simulink model "SIFT"  (R2015a)
settings: Solver=ode45  StartTime=0.0  StopTime=10.0  RelTol=1e-3
InitFcn:
  | %% DSPBuilder Start
  | alt_dspbuilder_update_model(bdroot)
  | %% DSPBuilder End
libraries: allblocks_alteradspbuilder2 x2272
(part 19 of 26)

== system SIFT/sift_octave1/get_descriptor/scale_space/Gaussian_scale4/Mul ==
  In00 : Inport
  In01 : Inport  Port=2
  In02 : Inport  Port=3
  In03 : Inport  Port=4
  In04 : Inport  Port=5
  In10 : Inport  Port=6
  In11 : Inport  Port=7
  In12 : Inport  Port=8
  In13 : Inport  Port=9
  In14 : Inport  Port=10
  In20 : Inport  Port=11
  In21 : Inport  Port=12
  In22 : Inport  Port=13
  In23 : Inport  Port=14
  In24 : Inport  Port=15
  In30 : Inport  Port=16
  In31 : Inport  Port=17
  In32 : Inport  Port=18
  In33 : Inport  Port=19
  In34 : Inport  Port=20
  In40 : Inport  Port=21
  In41 : Inport  Port=22
  In42 : Inport  Port=23
  In43 : Inport  Port=24
  In44 : Inport  Port=25
  clken : Inport  Port=26
  Delay : allblocks_alteradspbuilder2/Delay  pipeline=1  pipeline_display=1  ClockPhase=1  use_ena=on  use_sclr=off  allowFloatingPointOverride=on  logOutputs=off  logFile=C:\Users\ASUS\Desktop\sift_fpga\Octave_2\tb_SIFT\SIFT_sift%5Foctave1_get%5Fdescriptor_scale%5Fspace_Gaussian%5Fscale4_Mul_Delay.fixedpointlog  use_init=off  reset_value=1
  Delay1 : allblocks_alteradspbuilder2/Delay  pipeline=1  pipeline_display=1  ClockPhase=1  use_ena=on  use_sclr=off  allowFloatingPointOverride=on  logOutputs=off  logFile=C:\Users\ASUS\Desktop\sift_fpga\Octave_2\tb_SIFT\SIFT_sift%5Foctave1_get%5Fdescriptor_scale%5Fspace_Gaussian%5Fscale4_Mul_Delay1.fixedpointlog  use_init=off  reset_value=1
  Delay10 : allblocks_alteradspbuilder2/Delay  pipeline=1  pipeline_display=1  ClockPhase=1  use_ena=on  use_sclr=off  allowFloatingPointOverride=on  logOutputs=off  logFile=C:\Users\ASUS\Desktop\sift_fpga\Octave_2\tb_SIFT\SIFT_sift%5Foctave1_get%5Fdescriptor_scale%5Fspace_Gaussian%5Fscale4_Mul_Delay10.fixedpointlog  use_init=off  reset_value=1
  Delay11 : allblocks_alteradspbuilder2/Delay  pipeline=1  pipeline_display=1  ClockPhase=1  use_ena=on  use_sclr=off  allowFloatingPointOverride=on  logOutputs=off  logFile=C:\Users\ASUS\Desktop\sift_fpga\Octave_2\tb_SIFT\SIFT_sift%5Foctave1_get%5Fdescriptor_scale%5Fspace_Gaussian%5Fscale4_Mul_Delay11.fixedpointlog  use_init=off  reset_value=1
  Delay12 : allblocks_alteradspbuilder2/Delay  pipeline=1  pipeline_display=1  ClockPhase=1  use_ena=on  use_sclr=off  allowFloatingPointOverride=on  logOutputs=off  logFile=C:\Users\ASUS\Desktop\sift_fpga\Octave_2\tb_SIFT\SIFT_sift%5Foctave1_get%5Fdescriptor_scale%5Fspace_Gaussian%5Fscale4_Mul_Delay12.fixedpointlog  use_init=off  reset_value=1
  Delay13 : allblocks_alteradspbuilder2/Delay  pipeline=1  pipeline_display=1  ClockPhase=1  use_ena=on  use_sclr=off  allowFloatingPointOverride=on  logOutputs=off  logFile=C:\Users\ASUS\Desktop\sift_fpga\Octave_2\tb_SIFT\SIFT_sift%5Foctave1_get%5Fdescriptor_scale%5Fspace_Gaussian%5Fscale4_Mul_Delay13.fixedpointlog  use_init=off  reset_value=1
  Delay14 : allblocks_alteradspbuilder2/Delay  pipeline=1  pipeline_display=1  ClockPhase=1  use_ena=on  use_sclr=off  allowFloatingPointOverride=on  logOutputs=off  logFile=C:\Users\ASUS\Desktop\sift_fpga\Octave_2\tb_SIFT\SIFT_sift%5Foctave1_get%5Fdescriptor_scale%5Fspace_Gaussian%5Fscale4_Mul_Delay14.fixedpointlog  use_init=off  reset_value=1
  Delay15 : allblocks_alteradspbuilder2/Delay  pipeline=1  pipeline_display=1  ClockPhase=1  use_ena=on  use_sclr=off  allowFloatingPointOverride=on  logOutputs=off  logFile=C:\Users\ASUS\Desktop\sift_fpga\Octave_2\tb_SIFT\SIFT_sift%5Foctave1_get%5Fdescriptor_scale%5Fspace_Gaussian%5Fscale4_Mul_Delay15.fixedpointlog  use_init=off  reset_value=1
  Delay16 : allblocks_alteradspbuilder2/Delay  pipeline=1  pipeline_display=1  ClockPhase=1  use_ena=on  use_sclr=off  allowFloatingPointOverride=on  logOutputs=off  logFile=C:\Users\ASUS\Desktop\sift_fpga\Octave_2\tb_SIFT\SIFT_sift%5Foctave1_get%5Fdescriptor_scale%5Fspace_Gaussian%5Fscale4_Mul_Delay16.fixedpointlog  use_init=off  reset_value=1
  Delay17 : allblocks_alteradspbuilder2/Delay  pipeline=1  pipeline_display=1  ClockPhase=1  use_ena=on  use_sclr=off  allowFloatingPointOverride=on  logOutputs=off  logFile=C:\Users\ASUS\Desktop\sift_fpga\Octave_2\tb_SIFT\SIFT_sift%5Foctave1_get%5Fdescriptor_scale%5Fspace_Gaussian%5Fscale4_Mul_Delay17.fixedpointlog  use_init=off  reset_value=1
  Delay18 : allblocks_alteradspbuilder2/Delay  pipeline=1  pipeline_display=1  ClockPhase=1  use_ena=on  use_sclr=off  allowFloatingPointOverride=on  logOutputs=off  logFile=C:\Users\ASUS\Desktop\sift_fpga\Octave_2\tb_SIFT\SIFT_sift%5Foctave1_get%5Fdescriptor_scale%5Fspace_Gaussian%5Fscale4_Mul_Delay18.fixedpointlog  use_init=off  reset_value=1
  Delay19 : allblocks_alteradspbuilder2/Delay  pipeline=1  pipeline_display=1  ClockPhase=1  use_ena=on  use_sclr=off  allowFloatingPointOverride=on  logOutputs=off  logFile=C:\Users\ASUS\Desktop\sift_fpga\Octave_2\tb_SIFT\SIFT_sift%5Foctave1_get%5Fdescriptor_scale%5Fspace_Gaussian%5Fscale4_Mul_Delay19.fixedpointlog  use_init=off  reset_value=1
  Delay2 : allblocks_alteradspbuilder2/Delay  pipeline=1  pipeline_display=1  ClockPhase=1  use_ena=on  use_sclr=off  allowFloatingPointOverride=on  logOutputs=off  logFile=C:\Users\ASUS\Desktop\sift_fpga\Octave_2\tb_SIFT\SIFT_sift%5Foctave1_get%5Fdescriptor_scale%5Fspace_Gaussian%5Fscale4_Mul_Delay2.fixedpointlog  use_init=off  reset_value=1
  Delay20 : allblocks_alteradspbuilder2/Delay  pipeline=1  pipeline_display=1  ClockPhase=1  use_ena=on  use_sclr=off  allowFloatingPointOverride=on  logOutputs=off  logFile=C:\Users\ASUS\Desktop\sift_fpga\Octave_2\tb_SIFT\SIFT_sift%5Foctave1_get%5Fdescriptor_scale%5Fspace_Gaussian%5Fscale4_Mul_Delay20.fixedpointlog  use_init=off  reset_value=1
  Delay21 : allblocks_alteradspbuilder2/Delay  pipeline=1  pipeline_display=1  ClockPhase=1  use_ena=on  use_sclr=off  allowFloatingPointOverride=on  logOutputs=off  logFile=C:\Users\ASUS\Desktop\sift_fpga\Octave_2\tb_SIFT\SIFT_sift%5Foctave1_get%5Fdescriptor_scale%5Fspace_Gaussian%5Fscale4_Mul_Delay21.fixedpointlog  use_init=off  reset_value=1
  Delay22 : allblocks_alteradspbuilder2/Delay  pipeline=1  pipeline_display=1  ClockPhase=1  use_ena=on  use_sclr=off  allowFloatingPointOverride=on  logOutputs=off  logFile=C:\Users\ASUS\Desktop\sift_fpga\Octave_2\tb_SIFT\SIFT_sift%5Foctave1_get%5Fdescriptor_scale%5Fspace_Gaussian%5Fscale4_Mul_Delay22.fixedpointlog  use_init=off  reset_value=1
  Delay23 : allblocks_alteradspbuilder2/Delay  pipeline=1  pipeline_display=1  ClockPhase=1  use_ena=on  use_sclr=off  allowFloatingPointOverride=on  logOutputs=off  logFile=C:\Users\ASUS\Desktop\sift_fpga\Octave_2\tb_SIFT\SIFT_sift%5Foctave1_get%5Fdescriptor_scale%5Fspace_Gaussian%5Fscale4_Mul_Delay23.fixedpointlog  use_init=off  reset_value=1
  Delay24 : allblocks_alteradspbuilder2/Delay  pipeline=1  pipeline_display=1  ClockPhase=1  use_ena=on  use_sclr=off  allowFloatingPointOverride=on  logOutputs=off  logFile=C:\Users\ASUS\Desktop\sift_fpga\Octave_2\tb_SIFT\SIFT_sift%5Foctave1_get%5Fdescriptor_scale%5Fspace_Gaussian%5Fscale4_Mul_Delay24.fixedpointlog  use_init=off  reset_value=1
  Delay3 : allblocks_alteradspbuilder2/Delay  pipeline=1  pipeline_display=1  ClockPhase=1  use_ena=on  use_sclr=off  allowFloatingPointOverride=on  logOutputs=off  logFile=C:\Users\ASUS\Desktop\sift_fpga\Octave_2\tb_SIFT\SIFT_sift%5Foctave1_get%5Fdescriptor_scale%5Fspace_Gaussian%5Fscale4_Mul_Delay3.fixedpointlog  use_init=off  reset_value=1
  Delay4 : allblocks_alteradspbuilder2/Delay  pipeline=1  pipeline_display=1  ClockPhase=1  use_ena=on  use_sclr=off  allowFloatingPointOverride=on  logOutputs=off  logFile=C:\Users\ASUS\Desktop\sift_fpga\Octave_2\tb_SIFT\SIFT_sift%5Foctave1_get%5Fdescriptor_scale%5Fspace_Gaussian%5Fscale4_Mul_Delay4.fixedpointlog  use_init=off  reset_value=1
  Delay5 : allblocks_alteradspbuilder2/Delay  pipeline=1  pipeline_display=1  ClockPhase=1  use_ena=on  use_sclr=off  allowFloatingPointOverride=on  logOutputs=off  logFile=C:\Users\ASUS\Desktop\sift_fpga\Octave_2\tb_SIFT\SIFT_sift%5Foctave1_get%5Fdescriptor_scale%5Fspace_Gaussian%5Fscale4_Mul_Delay5.fixedpointlog  use_init=off  reset_value=1
  Delay6 : allblocks_alteradspbuilder2/Delay  pipeline=1  pipeline_display=1  ClockPhase=1  use_ena=on  use_sclr=off  allowFloatingPointOverride=on  logOutputs=off  logFile=C:\Users\ASUS\Desktop\sift_fpga\Octave_2\tb_SIFT\SIFT_sift%5Foctave1_get%5Fdescriptor_scale%5Fspace_Gaussian%5Fscale4_Mul_Delay6.fixedpointlog  use_init=off  reset_value=1
  Delay7 : allblocks_alteradspbuilder2/Delay  pipeline=1  pipeline_display=1  ClockPhase=1  use_ena=on  use_sclr=off  allowFloatingPointOverride=on  logOutputs=off  logFile=C:\Users\ASUS\Desktop\sift_fpga\Octave_2\tb_SIFT\SIFT_sift%5Foctave1_get%5Fdescriptor_scale%5Fspace_Gaussian%5Fscale4_Mul_Delay7.fixedpointlog  use_init=off  reset_value=1
  Delay8 : allblocks_alteradspbuilder2/Delay  pipeline=1  pipeline_display=1  ClockPhase=1  use_ena=on  use_sclr=off  allowFloatingPointOverride=on  logOutputs=off  logFile=C:\Users\ASUS\Desktop\sift_fpga\Octave_2\tb_SIFT\SIFT_sift%5Foctave1_get%5Fdescriptor_scale%5Fspace_Gaussian%5Fscale4_Mul_Delay8.fixedpointlog  use_init=off  reset_value=1
  Delay9 : allblocks_alteradspbuilder2/Delay  pipeline=1  pipeline_display=1  ClockPhase=1  use_ena=on  use_sclr=off  allowFloatingPointOverride=on  logOutputs=off  logFile=C:\Users\ASUS\Desktop\sift_fpga\Octave_2\tb_SIFT\SIFT_sift%5Foctave1_get%5Fdescriptor_scale%5Fspace_Gaussian%5Fscale4_Mul_Delay9.fixedpointlog  use_init=off  reset_value=1
  Gain : allblocks_alteradspbuilder2/Gain  vgain=0.0232  BusType=Unsigned Fractional  bwl=8  bwr=16  pipeline=16  pipeline_display=16  allowFloatingPointOverride=on  logOutputs=off  logFile=C:\Users\ASUS\Desktop\sift_fpga\Octave_2\tb_SIFT\SIFT_sift%5Foctave1_get%5Fdescriptor_scale%5Fspace_Gaussian%5Fscale4_Mul_Gain.fixedpointlog  use_ena=on  use_aclr=off  lpm=off  MaskValue=1
  Gain1 : allblocks_alteradspbuilder2/Gain  vgain=0.0338  BusType=Unsigned Fractional  bwl=8  bwr=16  pipeline=16  pipeline_display=16  allowFloatingPointOverride=on  logOutputs=off  logFile=C:\Users\ASUS\Desktop\sift_fpga\Octave_2\tb_SIFT\SIFT_sift%5Foctave1_get%5Fdescriptor_scale%5Fspace_Gaussian%5Fscale4_Mul_Gain1.fixedpointlog  use_ena=on  use_aclr=off  lpm=off  MaskValue=1
  Gain10 : allblocks_alteradspbuilder2/Gain  vgain=0.0383  BusType=Unsigned Fractional  bwl=8  bwr=16  pipeline=16  pipeline_display=16  allowFloatingPointOverride=on  logOutputs=off  logFile=C:\Users\ASUS\Desktop\sift_fpga\Octave_2\tb_SIFT\SIFT_sift%5Foctave1_get%5Fdescriptor_scale%5Fspace_Gaussian%5Fscale4_Mul_Gain10.fixedpointlog  use_ena=on  use_aclr=off  lpm=off  MaskValue=1
  Gain11 : allblocks_alteradspbuilder2/Gain  vgain=0.0558  BusType=Unsigned Fractional  bwl=8  bwr=16  pipeline=16  pipeline_display=16  allowFloatingPointOverride=on  logOutputs=off  logFile=C:\Users\ASUS\Desktop\sift_fpga\Octave_2\tb_SIFT\SIFT_sift%5Foctave1_get%5Fdescriptor_scale%5Fspace_Gaussian%5Fscale4_Mul_Gain11.fixedpointlog  use_ena=on  use_aclr=off  lpm=off  MaskValue=1
  Gain12 : allblocks_alteradspbuilder2/Gain  vgain=0.0632  BusType=Unsigned Fractional  bwl=8  bwr=16  pipeline=16  pipeline_display=16  allowFloatingPointOverride=on  logOutputs=off  logFile=C:\Users\ASUS\Desktop\sift_fpga\Octave_2\tb_SIFT\SIFT_sift%5Foctave1_get%5Fdescriptor_scale%5Fspace_Gaussian%5Fscale4_Mul_Gain12.fixedpointlog  use_ena=on  use_aclr=off  lpm=off  MaskValue=1
  Gain13 : allblocks_alteradspbuilder2/Gain  vgain=0.0558  BusType=Unsigned Fractional  bwl=8  bwr=16  pipeline=16  pipeline_display=16  allowFloatingPointOverride=on  logOutputs=off  logFile=C:\Users\ASUS\Desktop\sift_fpga\Octave_2\tb_SIFT\SIFT_sift%5Foctave1_get%5Fdescriptor_scale%5Fspace_Gaussian%5Fscale4_Mul_Gain13.fixedpointlog  use_ena=on  use_aclr=off  lpm=off  MaskValue=1
  Gain14 : allblocks_alteradspbuilder2/Gain  vgain=0.0383  BusType=Unsigned Fractional  bwl=8  bwr=16  pipeline=16  pipeline_display=16  allowFloatingPointOverride=on  logOutputs=off  logFile=C:\Users\ASUS\Desktop\sift_fpga\Octave_2\tb_SIFT\SIFT_sift%5Foctave1_get%5Fdescriptor_scale%5Fspace_Gaussian%5Fscale4_Mul_Gain14.fixedpointlog  use_ena=on  use_aclr=off  lpm=off  MaskValue=1
  Gain15 : allblocks_alteradspbuilder2/Gain  vgain=0.0338  BusType=Unsigned Fractional  bwl=8  bwr=16  pipeline=16  pipeline_display=16  allowFloatingPointOverride=on  logOutputs=off  logFile=C:\Users\ASUS\Desktop\sift_fpga\Octave_2\tb_SIFT\SIFT_sift%5Foctave1_get%5Fdescriptor_scale%5Fspace_Gaussian%5Fscale4_Mul_Gain15.fixedpointlog  use_ena=on  use_aclr=off  lpm=off  MaskValue=1
  Gain16 : allblocks_alteradspbuilder2/Gain  vgain=0.0492  BusType=Unsigned Fractional  bwl=8  bwr=16  pipeline=16  pipeline_display=16  allowFloatingPointOverride=on  logOutputs=off  logFile=C:\Users\ASUS\Desktop\sift_fpga\Octave_2\tb_SIFT\SIFT_sift%5Foctave1_get%5Fdescriptor_scale%5Fspace_Gaussian%5Fscale4_Mul_Gain16.fixedpointlog  use_ena=on  use_aclr=off  lpm=off  MaskValue=1
  Gain17 : allblocks_alteradspbuilder2/Gain  vgain=0.0558  BusType=Unsigned Fractional  bwl=8  bwr=16  pipeline=16  pipeline_display=16  allowFloatingPointOverride=on  logOutputs=off  logFile=C:\Users\ASUS\Desktop\sift_fpga\Octave_2\tb_SIFT\SIFT_sift%5Foctave1_get%5Fdescriptor_scale%5Fspace_Gaussian%5Fscale4_Mul_Gain17.fixedpointlog  use_ena=on  use_aclr=off  lpm=off  MaskValue=1
  Gain18 : allblocks_alteradspbuilder2/Gain  vgain=0.0492  BusType=Unsigned Fractional  bwl=8  bwr=16  pipeline=16  pipeline_display=16  allowFloatingPointOverride=on  logOutputs=off  logFile=C:\Users\ASUS\Desktop\sift_fpga\Octave_2\tb_SIFT\SIFT_sift%5Foctave1_get%5Fdescriptor_scale%5Fspace_Gaussian%5Fscale4_Mul_Gain18.fixedpointlog  use_ena=on  use_aclr=off  lpm=off  MaskValue=1
  Gain19 : allblocks_alteradspbuilder2/Gain  vgain=0.0338  BusType=Unsigned Fractional  bwl=8  bwr=16  pipeline=16  pipeline_display=16  allowFloatingPointOverride=on  logOutputs=off  logFile=C:\Users\ASUS\Desktop\sift_fpga\Octave_2\tb_SIFT\SIFT_sift%5Foctave1_get%5Fdescriptor_scale%5Fspace_Gaussian%5Fscale4_Mul_Gain19.fixedpointlog  use_ena=on  use_aclr=off  lpm=off  MaskValue=1
  Gain2 : allblocks_alteradspbuilder2/Gain  vgain=0.0383  BusType=Unsigned Fractional  bwl=8  bwr=16  pipeline=16  pipeline_display=16  allowFloatingPointOverride=on  logOutputs=off  logFile=C:\Users\ASUS\Desktop\sift_fpga\Octave_2\tb_SIFT\SIFT_sift%5Foctave1_get%5Fdescriptor_scale%5Fspace_Gaussian%5Fscale4_Mul_Gain2.fixedpointlog  use_ena=on  use_aclr=off  lpm=off  MaskValue=1
  Gain20 : allblocks_alteradspbuilder2/Gain  vgain=0.0232  BusType=Unsigned Fractional  bwl=8  bwr=16  pipeline=16  pipeline_display=16  allowFloatingPointOverride=on  logOutputs=off  logFile=C:\Users\ASUS\Desktop\sift_fpga\Octave_2\tb_SIFT\SIFT_sift%5Foctave1_get%5Fdescriptor_scale%5Fspace_Gaussian%5Fscale4_Mul_Gain20.fixedpointlog  use_ena=on  use_aclr=off  lpm=off  MaskValue=1
  Gain21 : allblocks_alteradspbuilder2/Gain  vgain=0.0338  BusType=Unsigned Fractional  bwl=8  bwr=16  pipeline=16  pipeline_display=16  allowFloatingPointOverride=on  logOutputs=off  logFile=C:\Users\ASUS\Desktop\sift_fpga\Octave_2\tb_SIFT\SIFT_sift%5Foctave1_get%5Fdescriptor_scale%5Fspace_Gaussian%5Fscale4_Mul_Gain21.fixedpointlog  use_ena=on  use_aclr=off  lpm=off  MaskValue=1
  Gain22 : allblocks_alteradspbuilder2/Gain  vgain=0.0383  BusType=Unsigned Fractional  bwl=8  bwr=16  pipeline=16  pipeline_display=16  allowFloatingPointOverride=on  logOutputs=off  logFile=C:\Users\ASUS\Desktop\sift_fpga\Octave_2\tb_SIFT\SIFT_sift%5Foctave1_get%5Fdescriptor_scale%5Fspace_Gaussian%5Fscale4_Mul_Gain22.fixedpointlog  use_ena=on  use_aclr=off  lpm=off  MaskValue=1
  Gain23 : allblocks_alteradspbuilder2/Gain  vgain=0.0338  BusType=Unsigned Fractional  bwl=8  bwr=16  pipeline=16  pipeline_display=16  allowFloatingPointOverride=on  logOutputs=off  logFile=C:\Users\ASUS\Desktop\sift_fpga\Octave_2\tb_SIFT\SIFT_sift%5Foctave1_get%5Fdescriptor_scale%5Fspace_Gaussian%5Fscale4_Mul_Gain23.fixedpointlog  use_ena=on  use_aclr=off  lpm=off  MaskValue=1
  Gain24 : allblocks_alteradspbuilder2/Gain  vgain=0.0232  BusType=Unsigned Fractional  bwl=8  bwr=16  pipeline=16  pipeline_display=16  allowFloatingPointOverride=on  logOutputs=off  logFile=C:\Users\ASUS\Desktop\sift_fpga\Octave_2\tb_SIFT\SIFT_sift%5Foctave1_get%5Fdescriptor_scale%5Fspace_Gaussian%5Fscale4_Mul_Gain24.fixedpointlog  use_ena=on  use_aclr=off  lpm=off  MaskValue=1
  Gain3 : allblocks_alteradspbuilder2/Gain  vgain=0.0338  BusType=Unsigned Fractional  bwl=8  bwr=16  pipeline=16  pipeline_display=16  allowFloatingPointOverride=on  logOutputs=off  logFile=C:\Users\ASUS\Desktop\sift_fpga\Octave_2\tb_SIFT\SIFT_sift%5Foctave1_get%5Fdescriptor_scale%5Fspace_Gaussian%5Fscale4_Mul_Gain3.fixedpointlog  use_ena=on  use_aclr=off  lpm=off  MaskValue=1
  Gain4 : allblocks_alteradspbuilder2/Gain  vgain=0.0232  BusType=Unsigned Fractional  bwl=8  bwr=16  pipeline=16  pipeline_display=16  allowFloatingPointOverride=on  logOutputs=off  logFile=C:\Users\ASUS\Desktop\sift_fpga\Octave_2\tb_SIFT\SIFT_sift%5Foctave1_get%5Fdescriptor_scale%5Fspace_Gaussian%5Fscale4_Mul_Gain4.fixedpointlog  use_ena=on  use_aclr=off  lpm=off  MaskValue=1
  Gain5 : allblocks_alteradspbuilder2/Gain  vgain=0.0338  BusType=Unsigned Fractional  bwl=8  bwr=16  pipeline=16  pipeline_display=16  allowFloatingPointOverride=on  logOutputs=off  logFile=C:\Users\ASUS\Desktop\sift_fpga\Octave_2\tb_SIFT\SIFT_sift%5Foctave1_get%5Fdescriptor_scale%5Fspace_Gaussian%5Fscale4_Mul_Gain5.fixedpointlog  use_ena=on  use_aclr=off  lpm=off  MaskValue=1
  Gain6 : allblocks_alteradspbuilder2/Gain  vgain=0.0492  BusType=Unsigned Fractional  bwl=8  bwr=16  pipeline=16  pipeline_display=16  allowFloatingPointOverride=on  logOutputs=off  logFile=C:\Users\ASUS\Desktop\sift_fpga\Octave_2\tb_SIFT\SIFT_sift%5Foctave1_get%5Fdescriptor_scale%5Fspace_Gaussian%5Fscale4_Mul_Gain6.fixedpointlog  use_ena=on  use_aclr=off  lpm=off  MaskValue=1
  Gain7 : allblocks_alteradspbuilder2/Gain  vgain=0.0558  BusType=Unsigned Fractional  bwl=8  bwr=16  pipeline=16  pipeline_display=16  allowFloatingPointOverride=on  logOutputs=off  logFile=C:\Users\ASUS\Desktop\sift_fpga\Octave_2\tb_SIFT\SIFT_sift%5Foctave1_get%5Fdescriptor_scale%5Fspace_Gaussian%5Fscale4_Mul_Gain7.fixedpointlog  use_ena=on  use_aclr=off  lpm=off  MaskValue=1
  Gain8 : allblocks_alteradspbuilder2/Gain  vgain=0.0492  BusType=Unsigned Fractional  bwl=8  bwr=16  pipeline=16  pipeline_display=16  allowFloatingPointOverride=on  logOutputs=off  logFile=C:\Users\ASUS\Desktop\sift_fpga\Octave_2\tb_SIFT\SIFT_sift%5Foctave1_get%5Fdescriptor_scale%5Fspace_Gaussian%5Fscale4_Mul_Gain8.fixedpointlog  use_ena=on  use_aclr=off  lpm=off  MaskValue=1
  Gain9 : allblocks_alteradspbuilder2/Gain  vgain=0.0338  BusType=Unsigned Fractional  bwl=8  bwr=16  pipeline=16  pipeline_display=16  allowFloatingPointOverride=on  logOutputs=off  logFile=C:\Users\ASUS\Desktop\sift_fpga\Octave_2\tb_SIFT\SIFT_sift%5Foctave1_get%5Fdescriptor_scale%5Fspace_Gaussian%5Fscale4_Mul_Gain9.fixedpointlog  use_ena=on  use_aclr=off  lpm=off  MaskValue=1
  Parallel Adder Subtractor : allblocks_alteradspbuilder2/Parallel Adder Subtractor  number_of_inputs=25  direction=+  use_pipeline=on  pipeline_display=5  phase_selection=1  use_ena=on  use_aclr=off  allowFloatingPointOverride=on  logOutputs=off  logFile=C:\Users\ASUS\Desktop\sift_fpga\Octave_2\tb_SIFT\SIFT_sift%5Foctave1_get%5Fdescriptor_scale%5Fspace_Gaussian%5Fscale4_Mul_Parallel+Adder+Subtractor.fixedpointlog
  pixel : Outport
  wires:
  In00/1 -> [data_00]
  In21/1 -> [data_21]
  In30/1 -> [data_30]
  In04/1 -> [data_04]
  In03/1 -> [data_03]
  In14/1 -> [data_14]
  In02/1 -> [data_02]
  In13/1 -> [data_13]
  In31/1 -> [data_31]
  In20/1 -> [data_20]
  In22/1 -> [data_22]
  In24/1 -> [data_24]
  In23/1 -> [data_23]
  In01/1 -> [data_01]
  In32/1 -> [data_32]
  In34/1 -> [data_34]
  In33/1 -> [data_33]
  In40/1 -> [data_40]
  In41/1 -> [data_41]
  In42/1 -> [data_42]
  In44/1 -> [data_44]
  In12/1 -> [data_12]
  In11/1 -> [data_11]
  In10/1 -> [data_10]
  Delay1/1 -> [mul_01]
  Delay4/1 -> [mul_04]
  [clken] -> Delay1/2, Gain1/2
  [data_11] -> Gain6/1
  Delay6/1 -> [mul_11]
  [data_12] -> Gain7/1
  [clken] -> Delay4/2, Gain4/2
  Delay2/1 -> [mul_02]
  [data_01] -> Gain1/1
  [data_04] -> Gain4/1
  Gain2/1 -> Delay2/1
  [clken] -> Delay6/2, Gain6/2
  Delay3/1 -> [mul_03]
  clken/1 -> [clken]
  [clken] -> Delay7/2, Gain7/2
  [data_02] -> Gain2/1
  Gain7/1 -> Delay7/1
  Gain1/1 -> Delay1/1
  [data_03] -> Gain3/1
  [data_00] -> Gain/1
  Gain5/1 -> Delay5/1
  Gain6/1 -> Delay6/1
  Delay5/1 -> [mul_10]
  Gain4/1 -> Delay4/1
  Gain/1 -> Delay/1
  Delay/1 -> [mul_00]
  [clken] -> Delay3/2, Gain3/2
  Gain3/1 -> Delay3/1
  [data_10] -> Gain5/1
  In43/1 -> [data_43]
  [clken] -> Delay2/2, Gain2/2
  [clken] -> Delay5/2, Gain5/2
  [clken] -> Delay13/2, Gain13/2
  [clken] -> Delay15/2, Gain15/2
  [data_22] -> Gain12/1
  [clken] -> Delay8/2, Gain8/2
  [data_20] -> Gain10/1
  [clken] -> Delay9/2, Gain9/2
  Delay9/1 -> [mul_14]
  Gain9/1 -> Delay9/1
  Delay10/1 -> [mul_20]
  [clken] -> Delay11/2, Gain11/2
  Delay11/1 -> [mul_21]
  [clken] -> Delay10/2, Gain10/2
  Gain10/1 -> Delay10/1
  Gain12/1 -> Delay12/1
  [data_14] -> Gain9/1
  Delay13/1 -> [mul_23]
  [clken] -> Delay14/2, Gain14/2
  Gain14/1 -> Delay14/1
  Delay7/1 -> [mul_12]
  [data_13] -> Gain8/1
  Gain15/1 -> Delay15/1
  [clken] -> Delay12/2, Gain12/2
  Gain13/1 -> Delay13/1
  Delay8/1 -> [mul_13]
  Delay12/1 -> [mul_22]
  [data_24] -> Gain14/1
  Gain11/1 -> Delay11/1
  [data_23] -> Gain13/1
  Delay14/1 -> [mul_24]
  Gain8/1 -> Delay8/1
  [data_30] -> Gain15/1
  [data_21] -> Gain11/1
  Gain18/1 -> Delay18/1
  Gain23/1 -> Delay23/1
  Gain16/1 -> Delay16/1
  Delay16/1 -> [mul_31]
  [data_34] -> Gain19/1
  [clken] -> Delay20/2, Gain20/2
  [clken] -> Delay19/2, Gain19/2
  Gain17/1 -> Delay17/1
  Delay17/1 -> [mul_32]
  Delay18/1 -> [mul_33]
  Gain20/1 -> Delay20/1
  Delay20/1 -> [mul_40]
  [clken] -> Delay17/2, Gain17/2
  [clken] -> Delay21/2, Gain21/2
  [data_31] -> Gain16/1
  [data_33] -> Gain18/1
  [clken] -> Delay16/2, Gain16/2
  Delay19/1 -> [mul_34]
  Gain21/1 -> Delay21/1
  [data_42] -> Gain22/1
  Delay21/1 -> [mul_41]
  Delay22/1 -> [mul_42]
  [data_43] -> Gain23/1
  [clken] -> Delay23/2, Gain23/2
  Delay15/1 -> [mul_30]
  [clken] -> Delay18/2, Gain18/2
  Gain19/1 -> Delay19/1
  Gain22/1 -> Delay22/1
  [data_40] -> Gain20/1
  [data_32] -> Gain17/1
  [data_41] -> Gain21/1
  [clken] -> Delay22/2, Gain22/2
  Delay24/1 -> [mul_44]
  Gain24/1 -> Delay24/1
  [clken] -> Delay24/2, Gain24/2
  [data_44] -> Gain24/1
  Delay23/1 -> [mul_43]
  [clken] -> Delay/2, Gain/2
  [pixel] -> pixel/1
  [mul_00] -> Parallel Adder Subtractor/1
  [mul_01] -> Parallel Adder Subtractor/2
  [mul_02] -> Parallel Adder Subtractor/3
  [mul_03] -> Parallel Adder Subtractor/4
  [mul_04] -> Parallel Adder Subtractor/5
  [mul_10] -> Parallel Adder Subtractor/6
  [mul_11] -> Parallel Adder Subtractor/7
  [mul_12] -> Parallel Adder Subtractor/8
  [mul_13] -> Parallel Adder Subtractor/9
  [mul_14] -> Parallel Adder Subtractor/10
  [mul_20] -> Parallel Adder Subtractor/11
  [mul_21] -> Parallel Adder Subtractor/12
  [mul_22] -> Parallel Adder Subtractor/13
  [mul_23] -> Parallel Adder Subtractor/14
  [mul_24] -> Parallel Adder Subtractor/15
  [mul_31] -> Parallel Adder Subtractor/17
  [mul_32] -> Parallel Adder Subtractor/18
  [mul_33] -> Parallel Adder Subtractor/19
  [mul_34] -> Parallel Adder Subtractor/20
  [mul_40] -> Parallel Adder Subtractor/21
  [mul_41] -> Parallel Adder Subtractor/22
  [mul_42] -> Parallel Adder Subtractor/23
  [mul_43] -> Parallel Adder Subtractor/24
  [mul_44] -> Parallel Adder Subtractor/25
  [mul_30] -> Parallel Adder Subtractor/16
  [clken] -> Parallel Adder Subtractor/26
  Parallel Adder Subtractor/1 -> [pixel]

== system SIFT/sift_octave1/get_descriptor/scale_space/Gaussian_scale4/line_buff ==
  dataIn : Inport
  clken : Inport  Port=2
  Delay : allblocks_alteradspbuilder2/Delay  pipeline=1  pipeline_display=1  ClockPhase=1  use_ena=on  use_sclr=off  allowFloatingPointOverride=on  logOutputs=off  logFile=C:\Users\ASUS\Desktop\sift_fpga\Octave_2\tb_SIFT\SIFT_sift%5Foctave1_get%5Fdescriptor_scale%5Fspace_Gaussian%5Fscale4_line%5Fbuff_Delay.fixedpointlog  use_init=off  reset_value=1
  Delay1 : allblocks_alteradspbuilder2/Delay  pipeline=1  pipeline_display=1  ClockPhase=1  use_ena=on  use_sclr=off  allowFloatingPointOverride=on  logOutputs=off  logFile=C:\Users\ASUS\Desktop\sift_fpga\Octave_2\tb_SIFT\SIFT_sift%5Foctave1_get%5Fdescriptor_scale%5Fspace_Gaussian%5Fscale4_line%5Fbuff_Delay1.fixedpointlog  use_init=off  reset_value=1
  Delay10 : allblocks_alteradspbuilder2/Delay  pipeline=1  pipeline_display=1  ClockPhase=1  use_ena=on  use_sclr=off  allowFloatingPointOverride=on  logOutputs=off  logFile=C:\Users\ASUS\Desktop\sift_fpga\Octave_2\tb_SIFT\SIFT_sift%5Foctave1_get%5Fdescriptor_scale%5Fspace_Gaussian%5Fscale4_line%5Fbuff_Delay10.fixedpointlog  use_init=off  reset_value=1
  Delay11 : allblocks_alteradspbuilder2/Delay  pipeline=1  pipeline_display=1  ClockPhase=1  use_ena=on  use_sclr=off  allowFloatingPointOverride=on  logOutputs=off  logFile=C:\Users\ASUS\Desktop\sift_fpga\Octave_2\tb_SIFT\SIFT_sift%5Foctave1_get%5Fdescriptor_scale%5Fspace_Gaussian%5Fscale4_line%5Fbuff_Delay11.fixedpointlog  use_init=off  reset_value=1
  Delay12 : allblocks_alteradspbuilder2/Delay  pipeline=1  pipeline_display=1  ClockPhase=1  use_ena=on  use_sclr=off  allowFloatingPointOverride=on  logOutputs=off  logFile=C:\Users\ASUS\Desktop\sift_fpga\Octave_2\tb_SIFT\SIFT_sift%5Foctave1_get%5Fdescriptor_scale%5Fspace_Gaussian%5Fscale4_line%5Fbuff_Delay12.fixedpointlog  use_init=off  reset_value=1
  Delay13 : allblocks_alteradspbuilder2/Delay  pipeline=1  pipeline_display=1  ClockPhase=1  use_ena=on  use_sclr=off  allowFloatingPointOverride=on  logOutputs=off  logFile=C:\Users\ASUS\Desktop\sift_fpga\Octave_2\tb_SIFT\SIFT_sift%5Foctave1_get%5Fdescriptor_scale%5Fspace_Gaussian%5Fscale4_line%5Fbuff_Delay13.fixedpointlog  use_init=off  reset_value=1
  Delay14 : allblocks_alteradspbuilder2/Delay  pipeline=1  pipeline_display=1  ClockPhase=1  use_ena=on  use_sclr=off  allowFloatingPointOverride=on  logOutputs=off  logFile=C:\Users\ASUS\Desktop\sift_fpga\Octave_2\tb_SIFT\SIFT_sift%5Foctave1_get%5Fdescriptor_scale%5Fspace_Gaussian%5Fscale4_line%5Fbuff_Delay14.fixedpointlog  use_init=off  reset_value=1
  Delay15 : allblocks_alteradspbuilder2/Delay  pipeline=1  pipeline_display=1  ClockPhase=1  use_ena=on  use_sclr=off  allowFloatingPointOverride=on  logOutputs=off  logFile=C:\Users\ASUS\Desktop\sift_fpga\Octave_2\tb_SIFT\SIFT_sift%5Foctave1_get%5Fdescriptor_scale%5Fspace_Gaussian%5Fscale4_line%5Fbuff_Delay15.fixedpointlog  use_init=off  reset_value=1
  Delay16 : allblocks_alteradspbuilder2/Delay  pipeline=1  pipeline_display=1  ClockPhase=1  use_ena=on  use_sclr=off  allowFloatingPointOverride=on  logOutputs=off  logFile=C:\Users\ASUS\Desktop\sift_fpga\Octave_2\tb_SIFT\SIFT_sift%5Foctave1_get%5Fdescriptor_scale%5Fspace_Gaussian%5Fscale4_line%5Fbuff_Delay16.fixedpointlog  use_init=off  reset_value=1
  Delay17 : allblocks_alteradspbuilder2/Delay  pipeline=1  pipeline_display=1  ClockPhase=1  use_ena=on  use_sclr=off  allowFloatingPointOverride=on  logOutputs=off  logFile=C:\Users\ASUS\Desktop\sift_fpga\Octave_2\tb_SIFT\SIFT_sift%5Foctave1_get%5Fdescriptor_scale%5Fspace_Gaussian%5Fscale4_line%5Fbuff_Delay17.fixedpointlog  use_init=off  reset_value=1
  Delay18 : allblocks_alteradspbuilder2/Delay  pipeline=1  pipeline_display=1  ClockPhase=1  use_ena=on  use_sclr=off  allowFloatingPointOverride=on  logOutputs=off  logFile=C:\Users\ASUS\Desktop\sift_fpga\Octave_2\tb_SIFT\SIFT_sift%5Foctave1_get%5Fdescriptor_scale%5Fspace_Gaussian%5Fscale4_line%5Fbuff_Delay18.fixedpointlog  use_init=off  reset_value=1
  Delay19 : allblocks_alteradspbuilder2/Delay  pipeline=1  pipeline_display=1  ClockPhase=1  use_ena=on  use_sclr=off  allowFloatingPointOverride=on  logOutputs=off  logFile=C:\Users\ASUS\Desktop\sift_fpga\Octave_2\tb_SIFT\SIFT_sift%5Foctave1_get%5Fdescriptor_scale%5Fspace_Gaussian%5Fscale4_line%5Fbuff_Delay19.fixedpointlog  use_init=off  reset_value=1
  Delay2 : allblocks_alteradspbuilder2/Delay  pipeline=1  pipeline_display=1  ClockPhase=1  use_ena=on  use_sclr=off  allowFloatingPointOverride=on  logOutputs=off  logFile=C:\Users\ASUS\Desktop\sift_fpga\Octave_2\tb_SIFT\SIFT_sift%5Foctave1_get%5Fdescriptor_scale%5Fspace_Gaussian%5Fscale4_line%5Fbuff_Delay2.fixedpointlog  use_init=off  reset_value=1
  Delay20 : allblocks_alteradspbuilder2/Delay  pipeline=1  pipeline_display=1  ClockPhase=1  use_ena=on  use_sclr=off  allowFloatingPointOverride=on  logOutputs=off  logFile=C:\Users\ASUS\Desktop\sift_fpga\Octave_2\tb_SIFT\SIFT_sift%5Foctave1_get%5Fdescriptor_scale%5Fspace_Gaussian%5Fscale4_line%5Fbuff_Delay20.fixedpointlog  use_init=off  reset_value=1
  Delay3 : allblocks_alteradspbuilder2/Delay  pipeline=1  pipeline_display=1  ClockPhase=1  use_ena=on  use_sclr=off  allowFloatingPointOverride=on  logOutputs=off  logFile=C:\Users\ASUS\Desktop\sift_fpga\Octave_2\tb_SIFT\SIFT_sift%5Foctave1_get%5Fdescriptor_scale%5Fspace_Gaussian%5Fscale4_line%5Fbuff_Delay3.fixedpointlog  use_init=off  reset_value=1
  Delay4 : allblocks_alteradspbuilder2/Delay  pipeline=1  pipeline_display=1  ClockPhase=1  use_ena=on  use_sclr=off  allowFloatingPointOverride=on  logOutputs=off  logFile=C:\Users\ASUS\Desktop\sift_fpga\Octave_2\tb_SIFT\SIFT_sift%5Foctave1_get%5Fdescriptor_scale%5Fspace_Gaussian%5Fscale4_line%5Fbuff_Delay4.fixedpointlog  use_init=off  reset_value=1
  Delay5 : allblocks_alteradspbuilder2/Delay  pipeline=1  pipeline_display=1  ClockPhase=1  use_ena=on  use_sclr=off  allowFloatingPointOverride=on  logOutputs=off  logFile=C:\Users\ASUS\Desktop\sift_fpga\Octave_2\tb_SIFT\SIFT_sift%5Foctave1_get%5Fdescriptor_scale%5Fspace_Gaussian%5Fscale4_line%5Fbuff_Delay5.fixedpointlog  use_init=off  reset_value=1
  Delay6 : allblocks_alteradspbuilder2/Delay  pipeline=1  pipeline_display=1  ClockPhase=1  use_ena=on  use_sclr=off  allowFloatingPointOverride=on  logOutputs=off  logFile=C:\Users\ASUS\Desktop\sift_fpga\Octave_2\tb_SIFT\SIFT_sift%5Foctave1_get%5Fdescriptor_scale%5Fspace_Gaussian%5Fscale4_line%5Fbuff_Delay6.fixedpointlog  use_init=off  reset_value=1
  Delay7 : allblocks_alteradspbuilder2/Delay  pipeline=1  pipeline_display=1  ClockPhase=1  use_ena=on  use_sclr=off  allowFloatingPointOverride=on  logOutputs=off  logFile=C:\Users\ASUS\Desktop\sift_fpga\Octave_2\tb_SIFT\SIFT_sift%5Foctave1_get%5Fdescriptor_scale%5Fspace_Gaussian%5Fscale4_line%5Fbuff_Delay7.fixedpointlog  use_init=off  reset_value=1
  Delay8 : allblocks_alteradspbuilder2/Delay  pipeline=1  pipeline_display=1  ClockPhase=1  use_ena=on  use_sclr=off  allowFloatingPointOverride=on  logOutputs=off  logFile=C:\Users\ASUS\Desktop\sift_fpga\Octave_2\tb_SIFT\SIFT_sift%5Foctave1_get%5Fdescriptor_scale%5Fspace_Gaussian%5Fscale4_line%5Fbuff_Delay8.fixedpointlog  use_init=off  reset_value=1
  Delay9 : allblocks_alteradspbuilder2/Delay  pipeline=1  pipeline_display=1  ClockPhase=1  use_ena=on  use_sclr=off  allowFloatingPointOverride=on  logOutputs=off  logFile=C:\Users\ASUS\Desktop\sift_fpga\Octave_2\tb_SIFT\SIFT_sift%5Foctave1_get%5Fdescriptor_scale%5Fspace_Gaussian%5Fscale4_line%5Fbuff_Delay9.fixedpointlog  use_init=off  reset_value=1
  Memory Delay : allblocks_alteradspbuilder2/Memory Delay  BusType=Unsigned Integer  bwl=8  bwr=0  pipeline=636  pipeline_display=636  ram_type=AUTO  use_ena=on  use_sclr=off  allowFloatingPointOverride=on  logOutputs=off  logFile=C:\Users\ASUS\Desktop\sift_fpga\Octave_2\tb_SIFT\SIFT_sift%5Foctave1_get%5Fdescriptor_scale%5Fspace_Gaussian%5Fscale4_line%5Fbuff_Memory+Delay.fixedpointlog
  Memory Delay1 : allblocks_alteradspbuilder2/Memory Delay  BusType=Unsigned Integer  bwl=8  bwr=0  pipeline=636  pipeline_display=636  ram_type=AUTO  use_ena=on  use_sclr=off  allowFloatingPointOverride=on  logOutputs=off  logFile=C:\Users\ASUS\Desktop\sift_fpga\Octave_2\tb_SIFT\SIFT_sift%5Foctave1_get%5Fdescriptor_scale%5Fspace_Gaussian%5Fscale4_line%5Fbuff_Memory+Delay1.fixedpointlog
  Memory Delay2 : allblocks_alteradspbuilder2/Memory Delay  BusType=Unsigned Integer  bwl=8  bwr=0  pipeline=636  pipeline_display=636  ram_type=AUTO  use_ena=on  use_sclr=off  allowFloatingPointOverride=on  logOutputs=off  logFile=C:\Users\ASUS\Desktop\sift_fpga\Octave_2\tb_SIFT\SIFT_sift%5Foctave1_get%5Fdescriptor_scale%5Fspace_Gaussian%5Fscale4_line%5Fbuff_Memory+Delay2.fixedpointlog
  Memory Delay3 : allblocks_alteradspbuilder2/Memory Delay  BusType=Unsigned Integer  bwl=8  bwr=0  pipeline=636  pipeline_display=636  ram_type=AUTO  use_ena=on  use_sclr=off  allowFloatingPointOverride=on  logOutputs=off  logFile=C:\Users\ASUS\Desktop\sift_fpga\Octave_2\tb_SIFT\SIFT_sift%5Foctave1_get%5Fdescriptor_scale%5Fspace_Gaussian%5Fscale4_line%5Fbuff_Memory+Delay3.fixedpointlog
  Out00 : Outport
  Out01 : Outport  Port=2
  Out02 : Outport  Port=3
  Out03 : Outport  Port=4
  Out04 : Outport  Port=5
  Out10 : Outport  Port=6
  Out11 : Outport  Port=7
  Out12 : Outport  Port=8
  Out13 : Outport  Port=9
  Out14 : Outport  Port=10
  Out20 : Outport  Port=11
  Out21 : Outport  Port=12
  Out22 : Outport  Port=13
  Out23 : Outport  Port=14
  Out24 : Outport  Port=15
  Out30 : Outport  Port=16
  Out31 : Outport  Port=17
  Out32 : Outport  Port=18
  Out33 : Outport  Port=19
  Out34 : Outport  Port=20
  Out40 : Outport  Port=21
  Out41 : Outport  Port=22
  Out42 : Outport  Port=23
  Out43 : Outport  Port=24
  Out44 : Outport  Port=25
  wires:
  [clken] -> Delay9/2
  [data_04] -> Out04/1
  [data_02] -> Out02/1
  [clken] -> Memory Delay1/2
  [data_44] -> Out44/1
  [data_33] -> Out33/1
  [clken] -> Delay4/2
  [clken] -> Delay11/2
  [data_32] -> Out32/1
  [data_31] -> Out31/1
  [data_40] -> Out40/1
  [data_43] -> Out43/1
  [data_42] -> Out42/1
  Delay11/1 -> [data_23], Delay12/1
  Memory Delay1/1 -> [data_20], Delay9/1
  [data_41] -> Out41/1
  Delay9/1 -> [data_21], Delay10/1
  [clken] -> Delay12/2
  [data_34] -> Out34/1
  [data_30] -> Out30/1
  Delay/1 -> [data_00], Delay1/1
  [clken] -> Delay1/2
  [clken] -> Delay/2
  [data_03] -> Out03/1
  [clken] -> Delay10/2
  Delay8/1 -> Memory Delay1/1, [data_14]
  Delay10/1 -> [data_22], Delay11/1
  [data_12] -> Out12/1
  dataIn/1 -> [data_in]
  Memory Delay3/1 -> [data_40], Delay20/1
  [clken] -> Memory Delay/2
  [clken] -> Delay2/2
  [data_22] -> Out22/1
  [clken] -> Delay14/2
  Delay17/1 -> [data_32], Delay18/1
  [clken] -> Delay20/2
  [data_10] -> Out10/1
  [data_21] -> Out21/1
  Delay12/1 -> [data_24], Memory Delay2/1
  Delay4/1 -> Memory Delay/1, [data_04]
  [clken] -> Delay3/2
  Delay2/1 -> [data_02], Delay3/1
  [clken] -> Memory Delay2/2
  [data_23] -> Out23/1
  [data_13] -> Out13/1
  clken/1 -> [clken]
  [data_11] -> Out11/1
  Delay18/1 -> [data_33], Delay19/1
  [data_20] -> Out20/1
  Delay1/1 -> [data_01], Delay2/1
  [data_24] -> Out24/1
  Memory Delay2/1 -> [data_30], Delay16/1
  [clken] -> Delay16/2
  [data_14] -> Out14/1
  [data_00] -> Out00/1
  [clken] -> Delay15/2
  [clken] -> Memory Delay3/2
  [data_01] -> Out01/1
  [data_in] -> Delay/1
  [clken] -> Delay7/2
  Delay19/1 -> Memory Delay3/1, [data_34]
  Delay14/1 -> [data_43], Delay15/1
  Memory Delay/1 -> [data_10], Delay5/1
  Delay5/1 -> [data_11], Delay6/1
  Delay16/1 -> [data_31], Delay17/1
  [clken] -> Delay6/2
  Delay6/1 -> [data_12], Delay7/1
  [clken] -> Delay13/2
  Delay3/1 -> [data_03], Delay4/1
  Delay15/1 -> [data_44]
  [clken] -> Delay18/2
  Delay13/1 -> [data_42], Delay14/1
  [clken] -> Delay5/2
  Delay7/1 -> [data_13], Delay8/1
  Delay20/1 -> [data_41], Delay13/1
  [clken] -> Delay17/2
  [clken] -> Delay19/2
  [clken] -> Delay8/2

== system SIFT/sift_octave1/matching/compare_descriptor/get_distance/BusSplitter ==
  data_in : Inport
  AltBus : allblocks_alteradspbuilder2/AltBus  BusType=Unsigned Integer  bwl=112  bwr=0  saturate=off  floatingPointInput=on  floatingPointOutput=on  logOutputs=off  logFile=C:\Users\ASUS\Desktop\sift_fpga\Octave_2\tb_SIFT\SIFT_sift%5Foctave1_matching_compare%5Fdescriptor_get%5Fdistance_BusSplitter_AltBus.fixedpointlog
  AltBus1 : allblocks_alteradspbuilder2/AltBus  BusType=Unsigned Integer  bwl=96  bwr=0  saturate=off  floatingPointInput=on  floatingPointOutput=on  logOutputs=off  logFile=C:\Users\ASUS\Desktop\sift_fpga\Octave_2\tb_SIFT\SIFT_sift%5Foctave1_matching_compare%5Fdescriptor_get%5Fdistance_BusSplitter_AltBus1.fixedpointlog
  AltBus10 : allblocks_alteradspbuilder2/AltBus  BusType=Unsigned Integer  bwl=16  bwr=0  saturate=off  floatingPointInput=on  floatingPointOutput=on  logOutputs=off  logFile=C:\Users\ASUS\Desktop\sift_fpga\Octave_2\tb_SIFT\SIFT_sift%5Foctave1_matching_compare%5Fdescriptor_get%5Fdistance_BusSplitter_AltBus10.fixedpointlog
  AltBus11 : allblocks_alteradspbuilder2/AltBus  BusType=Unsigned Integer  bwl=16  bwr=0  saturate=off  floatingPointInput=on  floatingPointOutput=on  logOutputs=off  logFile=C:\Users\ASUS\Desktop\sift_fpga\Octave_2\tb_SIFT\SIFT_sift%5Foctave1_matching_compare%5Fdescriptor_get%5Fdistance_BusSplitter_AltBus11.fixedpointlog
  AltBus12 : allblocks_alteradspbuilder2/AltBus  BusType=Unsigned Integer  bwl=16  bwr=0  saturate=off  floatingPointInput=on  floatingPointOutput=on  logOutputs=off  logFile=C:\Users\ASUS\Desktop\sift_fpga\Octave_2\tb_SIFT\SIFT_sift%5Foctave1_matching_compare%5Fdescriptor_get%5Fdistance_BusSplitter_AltBus12.fixedpointlog
  AltBus13 : allblocks_alteradspbuilder2/AltBus  BusType=Unsigned Integer  bwl=16  bwr=0  saturate=off  floatingPointInput=on  floatingPointOutput=on  logOutputs=off  logFile=C:\Users\ASUS\Desktop\sift_fpga\Octave_2\tb_SIFT\SIFT_sift%5Foctave1_matching_compare%5Fdescriptor_get%5Fdistance_BusSplitter_AltBus13.fixedpointlog
  AltBus2 : allblocks_alteradspbuilder2/AltBus  BusType=Unsigned Integer  bwl=80  bwr=0  saturate=off  floatingPointInput=on  floatingPointOutput=on  logOutputs=off  logFile=C:\Users\ASUS\Desktop\sift_fpga\Octave_2\tb_SIFT\SIFT_sift%5Foctave1_matching_compare%5Fdescriptor_get%5Fdistance_BusSplitter_AltBus2.fixedpointlog
  AltBus3 : allblocks_alteradspbuilder2/AltBus  BusType=Unsigned Integer  bwl=64  bwr=0  saturate=off  floatingPointInput=on  floatingPointOutput=on  logOutputs=off  logFile=C:\Users\ASUS\Desktop\sift_fpga\Octave_2\tb_SIFT\SIFT_sift%5Foctave1_matching_compare%5Fdescriptor_get%5Fdistance_BusSplitter_AltBus3.fixedpointlog
  AltBus4 : allblocks_alteradspbuilder2/AltBus  BusType=Unsigned Integer  bwl=48  bwr=0  saturate=off  floatingPointInput=on  floatingPointOutput=on  logOutputs=off  logFile=C:\Users\ASUS\Desktop\sift_fpga\Octave_2\tb_SIFT\SIFT_sift%5Foctave1_matching_compare%5Fdescriptor_get%5Fdistance_BusSplitter_AltBus4.fixedpointlog
  AltBus5 : allblocks_alteradspbuilder2/AltBus  BusType=Unsigned Integer  bwl=32  bwr=0  saturate=off  floatingPointInput=on  floatingPointOutput=on  logOutputs=off  logFile=C:\Users\ASUS\Desktop\sift_fpga\Octave_2\tb_SIFT\SIFT_sift%5Foctave1_matching_compare%5Fdescriptor_get%5Fdistance_BusSplitter_AltBus5.fixedpointlog
  AltBus6 : allblocks_alteradspbuilder2/AltBus  BusType=Unsigned Integer  bwl=16  bwr=0  saturate=off  floatingPointInput=on  floatingPointOutput=on  logOutputs=off  logFile=C:\Users\ASUS\Desktop\sift_fpga\Octave_2\tb_SIFT\SIFT_sift%5Foctave1_matching_compare%5Fdescriptor_get%5Fdistance_BusSplitter_AltBus6.fixedpointlog
  AltBus7 : allblocks_alteradspbuilder2/AltBus  BusType=Unsigned Integer  bwl=16  bwr=0  saturate=off  floatingPointInput=on  floatingPointOutput=on  logOutputs=off  logFile=C:\Users\ASUS\Desktop\sift_fpga\Octave_2\tb_SIFT\SIFT_sift%5Foctave1_matching_compare%5Fdescriptor_get%5Fdistance_BusSplitter_AltBus7.fixedpointlog
  AltBus8 : allblocks_alteradspbuilder2/AltBus  BusType=Unsigned Integer  bwl=16  bwr=0  saturate=off  floatingPointInput=on  floatingPointOutput=on  logOutputs=off  logFile=C:\Users\ASUS\Desktop\sift_fpga\Octave_2\tb_SIFT\SIFT_sift%5Foctave1_matching_compare%5Fdescriptor_get%5Fdistance_BusSplitter_AltBus8.fixedpointlog
  AltBus9 : allblocks_alteradspbuilder2/AltBus  BusType=Unsigned Integer  bwl=16  bwr=0  saturate=off  floatingPointInput=on  floatingPointOutput=on  logOutputs=off  logFile=C:\Users\ASUS\Desktop\sift_fpga\Octave_2\tb_SIFT\SIFT_sift%5Foctave1_matching_compare%5Fdescriptor_get%5Fdistance_BusSplitter_AltBus9.fixedpointlog
  Logical Bus Operator : allblocks_alteradspbuilder2/Logical Bus Operator  BusType=Unsigned Integer  bwl=128  bwr=0  LogicalOp_text=Shift Right  mask_value_num=-5  shift_amount=112  force_sign_ext=off  pipeline_display=0
  Logical Bus Operator1 : allblocks_alteradspbuilder2/Logical Bus Operator  BusType=Unsigned Integer  bwl=112  bwr=0  LogicalOp_text=Shift Right  mask_value_num=-5  shift_amount=96  force_sign_ext=off  pipeline_display=0
  Logical Bus Operator2 : allblocks_alteradspbuilder2/Logical Bus Operator  BusType=Unsigned Integer  bwl=96  bwr=0  LogicalOp_text=Shift Right  mask_value_num=-5  shift_amount=80  force_sign_ext=off  pipeline_display=0
  Logical Bus Operator3 : allblocks_alteradspbuilder2/Logical Bus Operator  BusType=Unsigned Integer  bwl=80  bwr=0  LogicalOp_text=Shift Right  mask_value_num=-5  shift_amount=64  force_sign_ext=off  pipeline_display=0
  Logical Bus Operator4 : allblocks_alteradspbuilder2/Logical Bus Operator  BusType=Unsigned Integer  bwl=64  bwr=0  LogicalOp_text=Shift Right  mask_value_num=-5  shift_amount=48  force_sign_ext=off  pipeline_display=0
  Logical Bus Operator5 : allblocks_alteradspbuilder2/Logical Bus Operator  BusType=Unsigned Integer  bwl=48  bwr=0  LogicalOp_text=Shift Right  mask_value_num=-5  shift_amount=32  force_sign_ext=off  pipeline_display=0
  Logical Bus Operator6 : allblocks_alteradspbuilder2/Logical Bus Operator  BusType=Unsigned Integer  bwl=32  bwr=0  LogicalOp_text=Shift Right  mask_value_num=-5  shift_amount=16  force_sign_ext=off  pipeline_display=0
  bin1 : Outport
  bin2 : Outport  Port=2
  bin3 : Outport  Port=3
  bin4 : Outport  Port=4
  bin5 : Outport  Port=5
  bin6 : Outport  Port=6
  bin7 : Outport  Port=7
  bin8 : Outport  Port=8
  wires:
  Logical Bus Operator6/1 -> AltBus7/1
  AltBus1/1 -> Logical Bus Operator2/1
  AltBus9/1 -> bin5/1
  AltBus8/1 -> bin6/1
  AltBus7/1 -> bin7/1
  AltBus6/1 -> bin8/1
  AltBus/1 -> Logical Bus Operator1/1
  AltBus10/1 -> bin4/1
  AltBus12/1 -> bin3/1
  AltBus11/1 -> bin1/1
  AltBus3/1 -> Logical Bus Operator4/1
  AltBus2/1 -> Logical Bus Operator3/1
  AltBus4/1 -> Logical Bus Operator5/1
  data_in/1 -> AltBus6/1, AltBus5/1, AltBus4/1, AltBus3/1, AltBus2/1, AltBus1/1, AltBus/1, Logical Bus Operator/1
  AltBus5/1 -> Logical Bus Operator6/1
  Logical Bus Operator1/1 -> AltBus13/1
  Logical Bus Operator2/1 -> AltBus12/1
  Logical Bus Operator/1 -> AltBus11/1
  Logical Bus Operator5/1 -> AltBus8/1
  Logical Bus Operator4/1 -> AltBus9/1
  Logical Bus Operator3/1 -> AltBus10/1
  AltBus13/1 -> bin2/1
